simulink model "injectorTestWax"  (R2020b)
settings: Solver=VariableStepAuto  StartTime=0.0  StopTime=10.0  RelTol=1e-3
libraries: fl_lib x9, nesl_utility x5
settings Model: Creator=abhin  LastModifiedBy=abhin

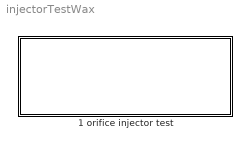
== system injectorTestWax ==
  1 orifice injector test : Subsystem  mask{upstreamPressure=40e5, injectorArea=1.6e-6, crossSection=0.1, dischargeCoeff=0.64}
      mask prompts: upstreamPressure "Upstream Pressure (Pa)"; injectorArea "Restriction Area (m^2)"; crossSection "Cross Sectional Area (m^2)"; dischargeCoeff "Discharge Coefficient"

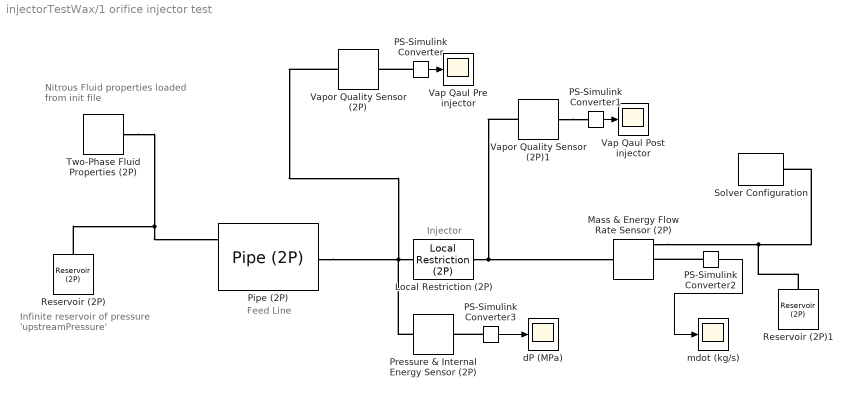
== system injectorTestWax/1 orifice injector test ==
  note: Injector
  note: Feed Line
  note: Nitrous Fluid properties loaded
      | from init file
  note: Infinite reservoir of pressure
      | 'upstreamPressure'
  Local Restriction (2P) : fl_lib/Two-Phase Fluid/Elements/Local Restriction (2P)  restriction_area=injectorArea m^2  area=crossSection m^2  Cd=dischargeCoeff  B_lam=0.999  mask(Local Restriction
(2P)){}
      settings: SourceProductBaseCode=SS  InternalSimscapePortConfiguration="{\"Bottom\":[],\"Left\":[{\"id\":\"A\",\"label\":\"A\",\"type\":\"foundation.two_phase_fluid.two_phase_fluid\"}],\"Right\":[{\"id\":\"B\",\"label\":\"B\",\"type\":\"foundation.two_phase_fluid.two_phase_fluid\"}],\"Top\":[]}"
  Mass & Energy Flow Rate Sensor (2P) : fl_lib/Two-Phase Fluid/Sensors/Mass & Energy Flow Rate Sensor (2P)
      settings: SourceProductBaseCode=SS  InternalSimscapePortConfiguration="{\"Bottom\":[],\"Left\":[{\"id\":\"A\",\"label\":\"A\",\"type\":\"foundation.two_phase_fluid.two_phase_fluid\"}],\"Right\":[{\"id\":\"B\",\"label\":\"B\",\"type\":\"foundation.two_phase_fluid.two_phase_fluid\"},{\"id\":\"M\",\"label\":\"M\",\"type\":\"output\"},{\"id\":\"PHI\",\"label\":\"Phi\",\"type\":\"output\"}],\"Top\":[]}"
  PS-Simulink Converter{,1..3} (4 alike) : nesl_utility/PS-Simulink Converter  PhysicalDomain=network_engine_domain  SubClassName=ps_output  LeftPortType=input  RightPortType=output  PseudoPeriodic=off  Frequencies=[]  Unit=inherit  AffineConversion=off
  Pipe (2P) : fl_lib/Two-Phase Fluid/Elements/Pipe (2P)  length=10 cm  area=1.96e-5 m^2  Dh=5e-3 m  length_add=10 cm  roughness=15e-6 m  Re_lam=2000  Re_tur=4000  shape_factor=64  Nu_lam=3.66  inertia=simscape.enum.onoff.on  energy_spec=foundation.enum.energy_spec.temperature  p_init=upstreamPressure Pa  T_init=293.15 K  x_init=0.5  alpha_init=0.5  h_init=1500 kJ/kg  u_init=1500 kJ/kg  mdot_init=0 kg/s  time_constant=0.1 s
      settings: SourceProductBaseCode=SS  InternalSimscapePortConfiguration="{\"Bottom\":[],\"Left\":[{\"id\":\"A\",\"label\":\"A\",\"type\":\"foundation.two_phase_fluid.two_phase_fluid\"},{\"id\":\"H\",\"label\":\"H\",\"type\":\"foundation.thermal.thermal\"}],\"Right\":[{\"id\":\"B\",\"label\":\"B\",\"type\":\"foundation.two_phase_fluid.two_phase_fluid\"}],\"Top\":[]}"
  Pressure & Internal Energy Sensor (2P) : fl_lib/Two-Phase Fluid/Sensors/Pressure & Internal Energy Sensor (2P)
      settings: SourceProductBaseCode=SS  InternalSimscapePortConfiguration="{\"Bottom\":[],\"Left\":[{\"id\":\"A\",\"label\":\"A\",\"type\":\"foundation.two_phase_fluid.two_phase_fluid\"}],\"Right\":[{\"id\":\"B\",\"label\":\"B\",\"type\":\"foundation.two_phase_fluid.two_phase_fluid\"},{\"id\":\"P\",\"label\":\"P\",\"type\":\"output\"},{\"id\":\"U\",\"label\":\"U\",\"type\":\"output\"}],\"Top\":[]}"
  Reservoir (2P) : fl_lib/Two-Phase Fluid/Elements/Reservoir (2P)  pressure_spec=foundation.enum.pressure_spec.specified  reservoir_pressure=upstreamPressure Pa  energy_spec=foundation.enum.energy_spec.quality  reservoir_temperature=293.15 K  reservoir_quality=0  reservoir_void_fraction=0.5  reservoir_enthalpy=1500 kJ/kg  reservoir_internal_energy=1500 kJ/kg  area_A=0.01 m^2
      settings: SourceProductBaseCode=SS
  Reservoir (2P)1 : fl_lib/Two-Phase Fluid/Elements/Reservoir (2P)  pressure_spec=foundation.enum.pressure_spec.atmospheric  reservoir_pressure=0.101325 MPa  energy_spec=foundation.enum.energy_spec.temperature  reservoir_temperature=293.15 K  reservoir_quality=0.5  reservoir_void_fraction=0.5  reservoir_enthalpy=1500 kJ/kg  reservoir_internal_energy=1500 kJ/kg  area_A=0.01 m^2
      settings: SourceProductBaseCode=SS
  Solver Configuration : nesl_utility/Solver Configuration  PhysicalDomain=network_engine_domain  SubClassName=solver  LeftPortType=input  RightPortType=generic  Tones=[]  Harmonics=[]  SimulateNoise=off  Profile=off  UseLocalSampling=off  EnableSwitchedLinearOptims=on  FrequencyDomain=off  UseCCode=off  RelTol=0.001  AbsTol=1e-06  MinStep=1e-09  ToWorkspace=off  RevertToSquareIcSolve=off  NumHomotopyIterations=100  PhasorMode=off  PhasorModeNumHarmonics=1  DoDC=off  ResidualTolerance=1e-09  UseLocalSolver=off  LocalSolverChoice=NE_BACKWARD_EULER_ADVANCER  LocalSolverSampleTime=0.001  DoFixedCost=off  MaxNonlinIter=3  MaxModeIter=2  ComputeImpulses=off  ImpulseIterations=2  LinearAlgebra=auto  EquationFormulation=NE_TIME_EF  DelaysMemoryBudget=1024  AutomaticFiltering=on  FilteringTimeConstant=0.001  PartitionStorageMethod=AS_NEEDED  PartitionMemoryBudget=1024  PartitionMethod=ROBUST
  Two-Phase Fluid Properties (2P) : fl_lib/Two-Phase Fluid/Utilities/Two-Phase Fluid Properties (2P)  u_min=sim.nitrousFluidTable.u_min kJ/kg  u_max=sim.nitrousFluidTable.u_max kJ/kg  unorm_liq=sim.nitrousFluidTable.liquid.unorm  unorm_vap=sim.nitrousFluidTable.vapor.unorm  p_TLU=sim.nitrousFluidTable.p MPa  v_liq=sim.nitrousFluidTable.liquid.v m^3/kg  v_vap=sim.nitrousFluidTable.vapor.v m^3/kg  s_liq=sim.nitrousFluidTable.liquid.s kJ/kg/K  s_vap=sim.nitrousFluidTable.vapor.s kJ/kg/K  T_liq=sim.nitrousFluidTable.liquid.T K  T_vap=sim.nitrousFluidTable.vapor.T K  nu_liq=sim.nitrousFluidTable.liquid.nu mm^2/s  nu_vap=sim.nitrousFluidTable.vapor.nu mm^2/s  k_liq=sim.nitrousFluidTable.liquid.k W/(m*K)  k_vap=sim.nitrousFluidTable.vapor.k W/(m*K)  Pr_liq=sim.nitrousFluidTable.liquid.Pr  Pr_vap=sim.nitrousFluidTable.vapor.Pr  u_sat_liq=sim.nitrousFluidTable.liquid.u_sat kJ/kg  u_sat_vap=sim.nitrousFluidTable.vapor.u_sat kJ/kg  p_crit=sim.nitrousFluidTable.p_crit MPa  critical_region=foundation.enum.critical_region.clip  p_crit_fraction=0.12  p_atm=0.101325 MPa  q_rev=0.01 Pa
      settings: SourceProductBaseCode=SS  InternalSimscapePortConfiguration="{\"Bottom\":[],\"Left\":[],\"Right\":[{\"id\":\"A\",\"label\":\"\",\"type\":\"foundation.two_phase_fluid.two_phase_fluid\"}],\"Top\":[]}"
  Vap Qaul Post injector : Scope
  Vap Qaul Pre injector : Scope
  Vapor Quality Sensor (2P) : fl_lib/Two-Phase Fluid/Sensors/Vapor Quality Sensor (2P)  vapor_fraction_spec=foundation.enum.vapor_fraction_spec.quality
      settings: SourceProductBaseCode=SS  InternalSimscapePortConfiguration="{\"Bottom\":[],\"Left\":[{\"id\":\"A\",\"label\":\"A\",\"type\":\"foundation.two_phase_fluid.two_phase_fluid\"}],\"Right\":[{\"id\":\"X\",\"label\":\"X\",\"type\":\"output\"}],\"Top\":[]}"
  Vapor Quality Sensor (2P)1 : fl_lib/Two-Phase Fluid/Sensors/Vapor Quality Sensor (2P)  vapor_fraction_spec=foundation.enum.vapor_fraction_spec.quality
      settings: SourceProductBaseCode=SS  InternalSimscapePortConfiguration="{\"Bottom\":[],\"Left\":[{\"id\":\"A\",\"label\":\"A\",\"type\":\"foundation.two_phase_fluid.two_phase_fluid\"}],\"Right\":[{\"id\":\"X\",\"label\":\"X\",\"type\":\"output\"}],\"Top\":[]}"
  dP (MPa) : Scope
  mdot (kg/s) : Scope
  wires:
  PS-Simulink Converter/1 -> Vap Qaul Pre injector/1
  PS-Simulink Converter2/1 -> mdot (kg/s)/1
  PS-Simulink Converter1/1 -> Vap Qaul Post injector/1
  PS-Simulink Converter3/1 -> dP (MPa)/1
  connections:
  Two-Phase Fluid Properties (2P)/RConn1 -- Reservoir (2P)/LConn1 -- Pipe (2P)/LConn1
  Pipe (2P)/RConn1 -- Local Restriction (2P)/LConn1 -- Vapor Quality Sensor (2P)/LConn1 -- Pressure & Internal Energy Sensor (2P)/LConn1
  Mass & Energy Flow Rate Sensor (2P)/RConn1 -- Solver Configuration/RConn1 -- Reservoir (2P)1/LConn1
  PS-Simulink Converter/LConn1 -- Vapor Quality Sensor (2P)/RConn1
  PS-Simulink Converter2/LConn1 -- Mass & Energy Flow Rate Sensor (2P)/RConn2
  Local Restriction (2P)/RConn1 -- Vapor Quality Sensor (2P)1/LConn1 -- Mass & Energy Flow Rate Sensor (2P)/LConn1
  Vapor Quality Sensor (2P)1/RConn1 -- PS-Simulink Converter1/LConn1
  PS-Simulink Converter3/LConn1 -- Pressure & Internal Energy Sensor (2P)/RConn2
